simulink library "mct"  (Simulink 8.1)
settings: Solver=ode1  StartTime=0.0  StopTime=Inf  FixedStep=0.001  RelTol=1e-3
PostLoadFcn:
  | , if any(exist('dsrtsu_mdlpostloadfcn', 'file') == [2, 3, 6]), try dsrtsu_mdlpostloadfcn('Execute', bdroot); catch fprintf('Error in PostLoadFcn (dsrtsu_mdlpostloadfcn) for model "%s":\n %s\n', bdroot, lasterr); end, end,
libraries: cms x1, ams x1, fms x1, vms_new x1
settings Model: DSRTSU_INTERNAL_RTI_VER=450  DSRTSU_INTERNAL_RTI_TYPE=rti1401  RTICANMMDATA=struct('GeneralSetupData',struct('modelroot','D:\ELN150201_TAIWAN\trunk\AdasDragon\software\sw_development\arch\app\ifo','generalsettings',struct('filesettings',struct('destfolder',struct('Name','RTICANMM_FILES','Check',1),'buildfolder',struct('Name','.','Check',1),'AbsDestfolder',struct('Name','D:\ELN150201_TAIWAN\trunk\AdasDragon\software\sw_development\arch\app\ifo\RTICANMM_FILES'),'AbsBuildfolder',struct('Name','D:\ELN150201_TAIWAN\trunk\AdasDragon\software\sw_development\arch\app\ifo'))),'options',struct('addpaths',1,'rmpaths',1,'addtrcexclusion',logical(1),'cannavigator',struct('checkmonitoring',0),'show_usrtrc',0,'use_usrtrc',0),'advanced',struct('options',[1 1 1 1 1 1 1 1 1 1 1 1 1 1 1 1 1 1 1 1 1 1 1 1 1 1 1 1 1 1 1 1 1 1 1 1 1 1 1 1 1 1 1 1 1 1 1 1 1 1 1 1 1 1 1 1 1 1 1 1 1 1 1 1 1 1 1 1 1 1 1 1 1 1 1 1 1 1 1 1 1 1 1 1 1 1 1 1 1 1 1 1 1 1 1 1 1 1 1 1]),'MPSetup',{{}},'modelname','mct','block','mct'))  DSRTSU_INTERNAL_RTIFPGA=40  Creator=tescamilla  LastModifiedBy=AT015555

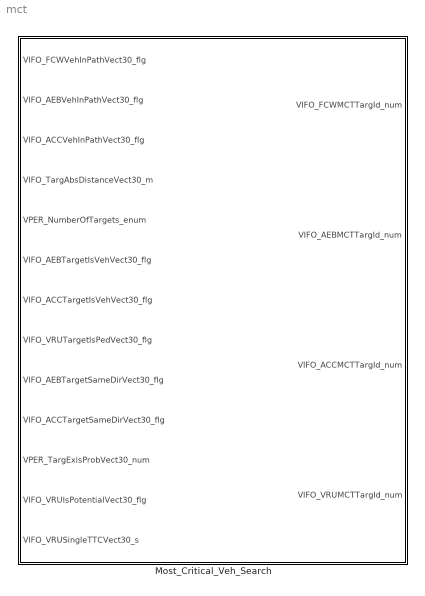
== system mct ==
  Most_Critical_Veh_Search : Subsystem  TreatAsAtomicUnit=on

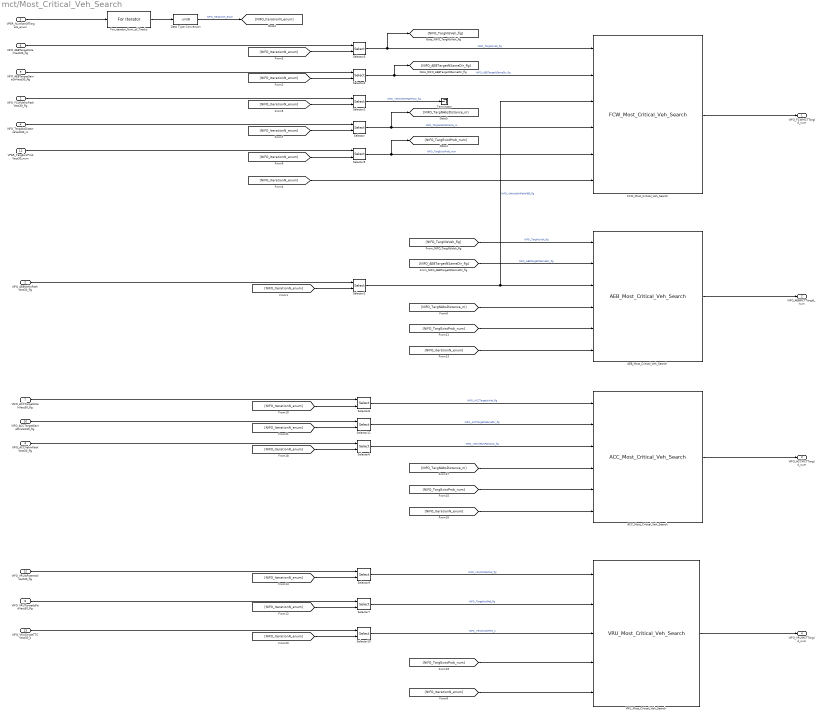
== system mct/Most_Critical_Veh_Search ==
  VIFO_FCWVehInPathVect30_flg : Inport
  VIFO_AEBVehInPathVect30_flg : Inport  Port=2
  VIFO_ACCVehInPathVect30_flg : Inport  Port=3
  VIFO_TargAbsDistanceVect30_m : Inport  Port=4
  VPER_NumberOfTargets_enum : Inport  Port=5
  VIFO_AEBTargetIsVehVect30_flg : Inport  Port=6
  VIFO_ACCTargetIsVehVect30_flg : Inport  Port=7
  VIFO_VRUTargetIsPedVect30_flg : Inport  Port=8
  VIFO_AEBTargetSameDirVect30_flg : Inport  Port=9
  VIFO_ACCTargetSameDirVect30_flg : Inport  Port=10
  VPER_TargExisProbVect30_num : Inport  Port=11
  VIFO_VRUIsPotentialVect30_flg : Inport  Port=12
  VIFO_VRUSingleTTCVect30_s : Inport  Port=13
  ACC_Most_Critical_Veh_Search : cms/ACC_Most_Critical_Veh_Search
  AEB_Most_Critical_Veh_Search : ams/AEB_Most_Critical_Veh_Search
  Data Type Conversion : DataTypeConversion  OutDataTypeStr=uint8
  FCW_Most_Critical_Veh_Search : fms/FCW_Most_Critical_Veh_Search
  For_iterator_Num_of_Tracks : ForIterator  ResetStates=reset  IterationSource=external  IterationVariableDataType=int8
  Selector{,1..11} (12 alike) : Selector  InputPortWidth=30  IndexOptions=Index vector (port)  Indices=[1 3]  OutputSizes=1
  Terminator : Terminator
  VRU_Most_Critical_Veh_Search : vms_new/VRU_Most_Critical_Veh_Search
  VIFO_FCWMCTTargId_num : Outport
  VIFO_AEBMCTTargId_num : Outport  Port=2
  VIFO_ACCMCTTargId_num : Outport  Port=3
  VIFO_VRUMCTTargId_num : Outport  Port=4
  wires:
  VRU_Most_Critical_Veh_Search/1 -> VIFO_VRUMCTTargId_num/1
  Selector10/1 -> VRU_Most_Critical_Veh_Search/3  "NIFO_VRUSimpleTTC_s"
  [NIFO_IterationN_enum] -> Selector10/2
  VIFO_VRUSingleTTCVect30_s/1 -> Selector10/1
  [NIFO_TargExistProb_num] -> VRU_Most_Critical_Veh_Search/4
  Selector9/1 -> VRU_Most_Critical_Veh_Search/1  "NIFO_VRUIsPotential_flg"
  [NIFO_IterationN_enum] -> Selector9/2
  VIFO_VRUIsPotentialVect30_flg/1 -> Selector9/1
  Selector7/1 -> VRU_Most_Critical_Veh_Search/2  "NIFO_TargetNIsPed_flg"
  [NIFO_IterationN_enum] -> Selector7/2
  VIFO_VRUTargetIsPedVect30_flg/1 -> Selector7/1
  [NIFO_IterationN_enum] -> VRU_Most_Critical_Veh_Search/5
  [NIFO_AEBTargetNSameDir_flg] -> AEB_Most_Critical_Veh_Search/2  "NIFO_AEBTargetNSameDir_flg"
  Selector4/1 -> FCW_Most_Critical_Veh_Search/2, [NIFO_AEBTargetNSameDir_flg]  "NIFO_AEBTargetNSameDir_flg"
  [NIFO_TargNIsVeh_flg] -> AEB_Most_Critical_Veh_Search/1  "NIFO_TargNIsVeh_flg"
  Selector3/1 -> FCW_Most_Critical_Veh_Search/1, [NIFO_TargNIsVeh_flg]  "NIFO_TargNIsVeh_flg"
  Data Type Conversion/1 -> [NIFO_IterationN_enum]  "NIFO_IterationN_enum"
  AEB_Most_Critical_Veh_Search/1 -> VIFO_AEBMCTTargId_num/1
  [NIFO_IterationN_enum] -> AEB_Most_Critical_Veh_Search/6
  [NIFO_TargNAbsDistance_m] -> AEB_Most_Critical_Veh_Search/4
  Selector1/1 -> FCW_Most_Critical_Veh_Search/3, AEB_Most_Critical_Veh_Search/3  "NIFO_VehicleNInPathAEB_flg"
  FCW_Most_Critical_Veh_Search/1 -> VIFO_FCWMCTTargId_num/1
  [NIFO_IterationN_enum] -> FCW_Most_Critical_Veh_Search/6
  Selector2/1 -> Terminator/1  "NIFO_VehicleNInPathFCW_flg"
  [NIFO_IterationN_enum] -> Selector1/2
  VIFO_AEBVehInPathVect30_flg/1 -> Selector1/1
  For_iterator_Num_of_Tracks/1 -> Data Type Conversion/1
  Selector/1 -> [NIFO_TargNAbsDistance_m], FCW_Most_Critical_Veh_Search/4  "NIFO_TargNAbsDistance_m"
  [NIFO_IterationN_enum] -> Selector/2
  [NIFO_IterationN_enum] -> Selector4/2
  VIFO_AEBTargetSameDirVect30_flg/1 -> Selector4/1
  [NIFO_IterationN_enum] -> Selector3/2
  VIFO_AEBTargetIsVehVect30_flg/1 -> Selector3/1
  [NIFO_IterationN_enum] -> Selector2/2
  VIFO_FCWVehInPathVect30_flg/1 -> Selector2/1
  VIFO_TargAbsDistanceVect30_m/1 -> Selector/1
  VPER_NumberOfTargets_enum/1 -> For_iterator_Num_of_Tracks/1
  VPER_TargExisProbVect30_num/1 -> Selector5/1
  [NIFO_IterationN_enum] -> Selector5/2
  Selector5/1 -> [NIFO_TargExistProb_num], FCW_Most_Critical_Veh_Search/5  "NIFO_TargExistProb_num"
  [NIFO_TargExistProb_num] -> AEB_Most_Critical_Veh_Search/5
  Selector8/1 -> ACC_Most_Critical_Veh_Search/1  "NIFO_ACCTargetIsVeh_flg"
  [NIFO_TargNAbsDistance_m] -> ACC_Most_Critical_Veh_Search/4
  [NIFO_TargExistProb_num] -> ACC_Most_Critical_Veh_Search/5
  [NIFO_IterationN_enum] -> ACC_Most_Critical_Veh_Search/6
  ACC_Most_Critical_Veh_Search/1 -> VIFO_ACCMCTTargId_num/1
  Selector6/1 -> ACC_Most_Critical_Veh_Search/3  "NIFO_VehicleNInPathACC_flg"
  [NIFO_IterationN_enum] -> Selector6/2
  VIFO_ACCVehInPathVect30_flg/1 -> Selector6/1
  [NIFO_IterationN_enum] -> Selector8/2
  VIFO_ACCTargetIsVehVect30_flg/1 -> Selector8/1
  [NIFO_IterationN_enum] -> Selector11/2
  VIFO_ACCTargetSameDirVect30_flg/1 -> Selector11/1
  Selector11/1 -> ACC_Most_Critical_Veh_Search/2  "NIFO_ACCTargetNSameDir_flg"
